simulink model "F16ASYM_Controlled"  (R2015a)
settings: Solver=ode3  SolverMode=SingleTasking  StartTime=0.0  StopTime=inf  FixedStep=T_sim  RelTol=1e-3
InitFcn:
  | load('NN_c_weights_Last_stable.mat')
StopFcn:
  | Final_results
values from neighbouring files (symbols this model uses):
  a1 = fitresult.p1    [Stall_protection.m]
  alpha_map_eval = ones(size(M_eval))*NaN    [Auto_trim_aid.m]    (also in Autotrim_maps.mat = [nan nan 0.277598136245 0.119432432992 0.0579479097061 0.027)
  beta_map_eval = ones(size(M_eval))*NaN    [Auto_trim_aid.m]    (also in Autotrim_maps.mat = [nan nan -0.00151549403324 0.00117807579006 -0.0052086799721)
  C_L_0 = fitresult.p2    [Stall_protection.m]
  G_eval = NaN*ones(size(M_sq,2),size(H_sq,2))    [Stall_protection.m]
  H_sq = unique(sort(H_sq))    [Stall_protection.m]
  H_sq_autotrim = min( F_envelope.H_1g):2000:max(F_envelope.H_1g)    [Auto_trim_aid.m]    (also in Autotrim_maps.mat = [0 2000 4000 6000 8000 10000 12000 14000 16000 18000])
  K_b_q_extrap_ACC = K_b_q_extrap    [RUN_ME.m]
  K_b_q_extrap_AoA = K_b_q_extrap    [RUN_ME.m]
  M_sq = unique(sort(M_sq))    [Stall_protection.m]
  M_sq_autotrim = 0:0.1:max(F_envelope.M_1g)    [Auto_trim_aid.m]    (also in Autotrim_maps.mat = [0 0.1 0.2 0.3 0.4 0.5 0.6 0.7 0.8 0.9 1 1.1 ... (21 element)
  T_sim = 0.02    [RUN_ME.m]
  tau_q_extrap_ACC = tau_q_extrap    [RUN_ME.m]
  tau_q_extrap_AoA = tau_q_extrap    [RUN_ME.m]
  velocity = M_eval(I,J)*a    [Auto_trim_aid.m]
undefined symbols (not defined in the file or in its folder): ACCEL, B, Earth, fi_flag_Simulink, GYRO, H_sq_sche, k_B, K_b_ACC_extrap, K_b_AoA_extrap, latitude, longitude, m, m_B, M_sq_sche, Model_used_flag, rad, s, sigbuilder_block, Stall_curve, tau_ACC_extrap, tau_AoA_extrap, Theta_1_roll_last, Theta_2_roll_last, Theta_3_roll_last, trim_control, trim_state, trim_throttle, V_Comp_A_w_z_last, V_Comp_last, V_Comp_last_ONE, V_long_lastA_w_z, V_long_lastAoA, V_roll_last, V_roll_lastMOD, V_yaw_last, W_Comp_A_w_z_last, W_Comp_last, W_long_lastA_w_z, W_long_lastAoA, W_roll_last, W_roll_lastMOD, W_yaw_last, WGS84
libraries: Adaptive_FaultTolerantControl x57, dspsigops x37, F16_Actuator_Library x14, commnoisgen2 x13, simulink x11, simulink_extras x10, dsparch4 x6, aerolibatmos2 x6, aerolibtransform2 x6, aerolibfltsims x3, dspvision x3, dspsnks4 x3
(part 2 of 14)

== system F16ASYM_Controlled/Plotting ==
  States : Inport
  Demmands : Inport  Port=2
  Control Defl : Inport  Port=3
  Ailerons : Scope  NumInputPorts=3
      settings: ShowLegends=on  TimeRange=25  YMin=0~0.04~-0.249  YMax=0.045~0.065~-0.231  SaveName=ScopeData6  Decimation=2
  Attitude : Scope  NumInputPorts=3
      settings: TimeRange=50  YMin=0.41~13.75~0.675  YMax=0.5~14.5~1.025  SaveName=EULER_PLOT  Decimation=2  SampleTime=0.001
  Demux : Demux  Outputs=5
  Demux1 : Demux  Outputs=20
  Demux2 : Demux  Outputs=7
  LEFs : Scope  NumInputPorts=2
      settings: ShowLegends=on  TimeRange=10  YMin=24.9965~-0.05  YMax=25.001~1.05  SaveName=ScopeData10  Decimation=2
  Load factors : Scope  NumInputPorts=3
      settings: YMin=-0.022~0.000572~0.999425  YMax=-0.0195~0.000579~0.999775  SaveName=ScopeData4  Decimation=20
  Mux{1..5} (5 alike) : Mux  Inputs=2
  Mux6 : Mux  Commented=on  Inputs=2
  Mux7 : Mux  Inputs=5
  Mux8 : Mux  Commented=on  Inputs=3
  "POW, Mach, q, ps" : Scope  NumInputPorts=4
      settings: YMin=-5~-5~-5~-5  YMax=5~5~5~5  SaveName=ScopeData5  Decimation=20
  Responses and commands : Scope  NumInputPorts=5
      settings: ShowLegends=on  TimeRange=50  YMin=1~11.6575~-0.04~-0.525~75  YMax=14~11.675~0.06~-0.325~125  SaveName=Responses  Decimation=2
  To Workspace : ToWorkspace  Commented=on  VariableName=DR1  SaveFormat=Timeseries  SampleTime=-1
  To Workspace1 : ToWorkspace  VariableName=Control_defl  SaveFormat=Timeseries  SampleTime=-1
  To Workspace2 : ToWorkspace  VariableName=Responses_out  SaveFormat=Timeseries  SampleTime=-1
  To Workspace3 : ToWorkspace  VariableName=ALL_Responses_out  SaveFormat=Timeseries  SampleTime=-1
  To Workspace4 : ToWorkspace  Commented=on  VariableName=SPPO4_ge  SaveFormat=Timeseries  SampleTime=-1
  To Workspace5 : ToWorkspace  Commented=on  VariableName=ROLL  SaveFormat=Timeseries  SampleTime=-1
  elevs : Scope  NumInputPorts=2
      settings: ShowLegends=on  TimeRange=10  YMin=-2.7018~-2.678  YMax=-2.6998~-2.67525  SaveName=ScopeData9  Decimation=2
  p,q,r : Scope  NumInputPorts=3
      settings: TimeRange=15  YMin=-3~-0.04~-3  YMax=7~0.04~9  SaveName=ScopeData3  Decimation=2
  position and altitude : Scope  NumInputPorts=3
      settings: YMin=12100~6e-11~13235  YMax=13700~8.75e-11~13320  Decimation=20
  wires:
  Demux1/1 -> position and altitude/1  "npos   (m)"
  Demux1/2 -> position and altitude/2  "epos   (m)"
  Demux1/3 -> position and altitude/3  "alt   (m)"
  Demux1/5 -> Attitude/2  "theta   (deg)"
  Demux1/6 -> Attitude/3  "psi  (deg)"
  Demux1/7 -> Mux5/2  "TAS   (m/s)"
  Demux1/8 -> Mux1/2  "alpha( deg)"
  Demux1/9 -> Mux3/2  "beta  (deg)"
  Demux1/10 -> To Workspace5/1, Mux6/1, p,q,r/1, Mux2/2  "p   (deg/s)"
  Demux1/11 -> Mux8/3, p,q,r/2  "q   (deg/s)"
  Demux1/12 -> Mux6/2, p,q,r/3  "r   (deg/s)"
  Demux1/14 -> Load factors/1  "nx (g)"
  Demux1/15 -> Load factors/2  "ny (g)"
  Demux1/16 -> Load factors/3  "nz (g)"
  Demux1/4 -> Attitude/1  "phi   (deg)"
  Demux1/17 -> "POW, Mach, q, ps"/2  "mach"
  Demux1/18 -> "POW, Mach, q, ps"/3  "qbar (Pa"
  Demux1/19 -> "POW, Mach, q, ps"/4  "ps (Pa)"
  States/1 -> To Workspace3/1, Demux1/1
  Demux1/13 -> "POW, Mach, q, ps"/1  "pow"
  Demmands/1 -> Demux/1
  Mux2/1 -> Mux7/3, Responses and commands/3
  Mux3/1 -> Mux7/4, Responses and commands/4
  Demux/2 -> Mux1/1  "alpha comm"
  Demux/3 -> Mux2/1  "p comm"
  Demux/4 -> Mux3/1  "beta comm"
  Mux4/1 -> Mux8/1, Mux7/1, Responses and commands/1
  Demux/1 -> Mux4/1  "A_w_z comm"
  Demux1/20 -> Mux4/2  "A_w_z (m/s^2)"
  Control Defl/1 -> To Workspace1/1, Demux2/1
  Demux2/3 -> Ailerons/1  "Aileron Left"
  Demux2/7 -> LEFs/2  "LEF Right"
  Demux2/6 -> LEFs/1  "LEF Left"
  Demux2/2 -> elevs/2  "Elevator_ Right"
  Demux2/5 -> Ailerons/3  "Rudder"
  Demux2/4 -> Ailerons/2  "Aielron Right"
  Mux5/1 -> Mux7/5, Responses and commands/5
  Demux/5 -> Mux5/1  "TAS comm"
  Mux1/1 -> Mux8/2, Mux7/2, Responses and commands/2
  Mux6/1 -> To Workspace/1
  Demux2/1 -> elevs/1  "Elevator_ Left"
  Mux7/1 -> To Workspace2/1
  Mux8/1 -> To Workspace4/1

== system F16ASYM_Controlled/Primary Controller ==
  A_w_z des : Inport
  AoA des (rad) : Inport  Port=2
  p des (rad/s) : Inport  Port=3
  beta des (rad) : Inport  Port=4
  Anti-windup A_w_z : Inport  Port=5
  Anti-windup AoA : Inport  Port=6
  Anti-windup beta : Inport  Port=7
  All measures : Inport  Port=8
  Anti-windup signals : Inport  Port=9
  P con  + Crossed NN + AWU+Lim + hand-over+Scheduling : Subsystem  VariantControl=Adaptive Controller Crossed+AWU+Lim+hand-over+Sched
  P con + Crossed NN + AWU+Lim + hand-over : Subsystem  VariantControl=Adaptive Controller Crossed+AWU+Lim+hand-over
  P con + adaptive Crossed NN + AWU+Lim + Scheduling : Subsystem  VariantControl=Adaptive Controller Crossed+AWU+Lim+Sched
  "P cont + adaptive Crossed NN + AWU+Lim " : Subsystem  VariantControl=Adaptive Controller Crossed+AWU+Lim
  P cont + adaptive Crossed NN + AWU+Lim ONELAYER : Subsystem  VariantControl=ONE
  P controller : Subsystem  VariantControl=P Controller
  P controller + adaptive Crossed NN : Subsystem  VariantControl=Adaptive Controller Crossed
  P controller + adaptive Isolated NN : Subsystem  VariantControl=Adaptive Controller Isolated
  PI Primary Controller : Subsystem  VariantControl=PI Controller
  Angular acc des : Outport
  Control_in : Outport  Port=2

== system F16ASYM_Controlled/SI and FDI ==
  Inexistent Reconfig bus : Inport
  Control comms : Inport  Port=2
  All  meas : Inport  Port=3
  SI and FDI: Realistic : Subsystem  VariantControl=Realistic
  SI and FDI: Unrealistic : Subsystem  VariantControl=Unrealistic
  Est reconf params : Outport

== system F16ASYM_Controlled/Sensors and filtering ==
  state : Inport
  Sensors and filtering. No noise : Subsystem  VariantControl=No noise
  Sensors and filtering. Noise : Subsystem  VariantControl=Noise
  All_measures : Outport

== system F16ASYM_Controlled/Signal Builder ==
  Demux : Demux  Tag=STV Demux  Outputs=1
  FromWs : FromWorkspace  Tag=STV FromWs  VariableName=tuvar  SampleTime=0
      SigBuilderData=|
      | common.afterFinalStr = 'Extrapolate'
      | common.sampleTime = 0
      | dataSet.timeRange = [0 10]
      | dataSet.name = 'Group 1'
      | sbobj.Groups.Name = 'Group 1'
      | sbobj.Groups.Signals.Name = 'Signal 1'
      | sbobj.Groups.Signals.XData = [0 8 8 8.5 8.5 10]
      | sbobj.Groups.Signals.YData = [0 0 0.51 0.51 0 0]
  Signal 1 : Outport  Tag=STV Outport
  wires:
  Demux/1 -> Signal 1/1
  FromWs/1 -> Demux/1

== system F16ASYM_Controlled/Speed-Throttle control ==
  All meas : Inport
  Throttle comm : Inport  Port=2
  delta TAS comm : Inport  Port=3
  "   " : Sum  Inputs=++|
  Add1 : Sum  Inputs=++|
  Manual Switch : ManualSwitch  CurrentSetting=0
  Stall protection TAS : Subsystem
  Throttle Trim Setting : Constant  Value=trim_throttle
  Throttle controller : Subsystem
  V_TAS des : Constant  Value=velocity
  Throttle des : Outport
  TAS des : Outport  Port=2
  wires:
  Throttle controller/1(Throttle des) -> Manual Switch/2
  Add1/1 -> Manual Switch/1
  Throttle Trim Setting/1 -> Add1/1
  Manual Switch/1 -> Throttle des/1
  Stall protection TAS/1(TAS des) -> Throttle controller/1(V_TAS des), TAS des/1
  Throttle comm/1 -> Add1/2
  delta TAS comm/1 -> "   "/2
  V_TAS des/1 -> "   "/1
  "   "/1 -> Stall protection TAS/1(TAS comm)
  All meas/1 -> Stall protection TAS/2(All meas), Throttle controller/2(All meas)

== system F16ASYM_Controlled/Stall protection A_z and AoA ==
  Control in : Inport
  Reconf param : Inport  Port=2
  All meas : Inport  Port=3
  A_w_z comm : Inport  Port=4
  AoA comm : Inport  Port=5
  AoA and load factor map : Subsystem  VariantControl=AoA and load factor
  Using AoA : Subsystem  VariantControl=Using AoA
  A_w_z des : Outport
  AoA des : Outport  Port=2

== system F16ASYM_Controlled/SubSystem3 ==

== system F16ASYM_Controlled/rad2deg ==
  note: npos,epos,alt
  note: phi
  note: theta
  note: psi
  note: v
  note: alpha
  note: beta
  note: p
  note: q
  note: r
  Params bus : Inport
  States Bus : Inport  Port=2
  Bus Selector : BusSelector  OutputSignals=States_out,Other outs
  Bus Selector1 : BusSelector  OutputSignals=A_w_CG
  Demux1 : Demux  Outputs=[3 1 1 1 1 1 1 1 1 1 1 3 3]
  Gain : Gain  Gain=-1
  Mux : Mux  Inputs=[3 1 1 1 1 1 1 1 1 1 1 3 3 1]
  Mux1 : Mux  Inputs=2
  Selector : Selector  InputPortWidth=3  Indices=3
  r2d{,1..7} (8 alike) : Gain  Gain=180/pi  SaturateOnIntegerOverflow=on  OutDataTypeStr=Inherit: Same as input  ParamDataTypeStr=Inherit: Same as input
  Out1 : Outport
  wires:
  Mux1/1 -> Demux1/1
  Demux1/2 -> r2d/1
  Demux1/3 -> r2d1/1
  Demux1/4 -> r2d2/1
  Demux1/1 -> Mux/1
  Demux1/5 -> Mux/5
  r2d2/1 -> Mux/4
  r2d1/1 -> Mux/3
  r2d/1 -> Mux/2
  Demux1/6 -> r2d3/1
  Demux1/7 -> r2d4/1
  Demux1/8 -> r2d5/1
  Demux1/9 -> r2d6/1
  Demux1/10 -> r2d7/1
  r2d4/1 -> Mux/7
  r2d5/1 -> Mux/8
  r2d6/1 -> Mux/9
  r2d7/1 -> Mux/10
  Mux/1 -> Out1/1
  Demux1/12 -> Mux/12  "nx,ny,nz"
  Demux1/13 -> Mux/13  "mach,qbar,ps"
  r2d3/1 -> Mux/6
  Demux1/11 -> Mux/11  "pow"
  Bus Selector/1 -> Mux1/1  "<States_out>"
  Bus Selector/2 -> Mux1/2  "<Other outs>"
  States Bus/1 -> Bus Selector/1
  Params bus/1 -> Bus Selector1/1
  Bus Selector1/1 -> Selector/1  "<A_w_CG>"
  Selector/1 -> Gain/1
  Gain/1 -> Mux/14

== system F16ASYM_Controlled/Anti-windup Calculation/Anti-windup: NO reconfigurable ==
  note: Reached Angular accel
  note: Converto to Angular accelerations
  Ang accel comm : Inport
  Est reconf : Inport  Port=2
  All_meas : Inport  Port=3
  Surf saturated : Inport  Port=4
  Control_defl : Inport  Port=5
  Analog Filter Design1 : dsparch4/Analog Filter Design  method=Butterworth  filttype=Lowpass  N=8  Wlo=2*pi/T_sim/4  Whi=80  Rp=2  Rs=40
  Analog Filter Design2 : dsparch4/Analog Filter Design  method=Butterworth  filttype=Lowpass  N=8  Wlo=2*pi/T_sim/4  Whi=80  Rp=2  Rs=40
  Analog Filter Design3 : dsparch4/Analog Filter Design  method=Butterworth  filttype=Lowpass  N=8  Wlo=2*pi/T_sim/4  Whi=80  Rp=2  Rs=40
  Ang Accel : MATLAB Function
  Antiwindup calculation : MATLAB Function  TreatAsAtomicUnit=on
  Bus Selector : BusSelector  OutputSignals=signal1.Alt meas (m),signal1.V_TAS (m/s),signal1.AoA meas (rad),signal1.SS meas (rad),signal1.omega_b meas (rad/s),signal1.Throttle_meas
  Bus Selector1 : BusSelector  OutputSignals=signal2.q (Pa),signal1.omega_b meas (rad/s)
  Demux : Demux  Outputs=3
  Demux1 : Demux  Outputs=3
  Effectiveness Matrix B : Constant  Value=B
  Memory1 : Memory  X0=[0,0,0]
  Mom coefficients that was reached : MATLABFcn  MATLABFcn=Moms_Coeff_estimator  OutputDimensions=3  OutputSignalType=real
  Moments : Subsystem
  Mux : Mux  Inputs=3
  Mux1 : Mux  Inputs=7
  Mux2 : Mux  Inputs=3
  Selector : Selector  InputPortWidth=8  Indices=1:7
  Terminator1 : Terminator
  Anti-windup signals : Outport
  wires:
  Selector/1 -> Antiwindup calculation/5(deflections), Mux1/7
  Mux1/1 -> Mom coefficients that was reached/1
  Bus Selector/5 -> Mux1/5  "<omega_b meas (rad/s)>"
  Bus Selector/1 -> Mux1/1  "<Alt meas (m)>"
  Bus Selector/2 -> Mux1/2  "<V_TAS (m/s)>"
  Bus Selector/3 -> Mux1/3  "<AoA meas (rad)>"
  Bus Selector/4 -> Mux1/4  "<SS meas (rad)>"
  Control_defl/1 -> Selector/1
  Bus Selector/6 -> Mux1/6  "<Throttle_meas>"
  Ang Accel/2(q_dot) -> Mux/2
  Ang Accel/3(r_dot) -> Mux/3
  Ang Accel/1(p_dot) -> Mux/1
  Bus Selector1/2 -> Ang Accel/4(omega_b)  "<omega_b meas (rad/s)>"
  Moments/3(N) -> Ang Accel/3(N)
  Moments/2(M) -> Ang Accel/2(M)
  Moments/1(L) -> Ang Accel/1(L)
  Bus Selector1/1 -> Moments/4(q)  "<q (Pa)>"
  Demux/3 -> Moments/3(C_N)
  Demux/2 -> Moments/2(C_M)
  Demux/1 -> Moments/1(C_L)
  Mom coefficients that was reached/1 -> Demux/1
  All_meas/1 -> Bus Selector/1, Bus Selector1/1
  Est reconf/1 -> Terminator1/1
  Mux/1 -> Antiwindup calculation/2(Ang_acell_achieved)
  Effectiveness Matrix B/1 -> Antiwindup calculation/4(B)
  Surf saturated/1 -> Antiwindup calculation/3(Saturations)
  Ang accel comm/1 -> Memory1/1
  Memory1/1 -> Antiwindup calculation/1(Ang_acell_comm)
  Mux2/1 -> Anti-windup signals/1
  Antiwindup calculation/1(AWU) -> Demux1/1
  Demux1/1 -> Analog Filter Design3/1
  Demux1/2 -> Analog Filter Design1/1
  Analog Filter Design3/1 -> Mux2/1
  Analog Filter Design1/1 -> Mux2/2
  Analog Filter Design2/1 -> Mux2/3
  Demux1/3 -> Analog Filter Design2/1

== system F16ASYM_Controlled/Anti-windup Calculation/Anti-windup: Reconfigurable ==
  note: INPUTS
      | States:
      |
      | 1. Altitude
      | 2. TAS velocity
      | 3. alpha in rad
      | 4. beta in rads
      | 5. P
      | 6. Q
      | 7. R
      | 8. Throttle
      | 9. Elevator_L in deg
      | 10. Elevator_R in deg
      | 11. Aileron_L
      | 12. Aileron_R
      | 13. Rudder
      | 14. LEF_L
      | 15. LEF_R
      |
      | RECONFIGURATION PARAMETERS
      |
      | 16. mass  Estimated mass
      | 17. S_current_L
      | 18. S_current_R
      | 19. S_fin_current
      | 20. x_cg
      | 21. Jy
      | 22. Jxz
      | 23. Jz
      | 24. Jx
      | 25. EFF_el_L
      | 26. EFF_el_R
      | 27. EFF_ail_L
      | 28 EFF_ail_R
      | 29. EFF_rud
      | 30. EFF_lef_L
      | 31. EFF_lef_R
      | 32. Delta_C_Lift_X
      | 33. Delta_C_Drag_X
      | 34. Delta_C_m_X
  note: Reached Angular accel
  note: Converto to Angular accelerations
  Ang accel comm : Inport
  Est reconf : Inport  Port=2
  All_meas : Inport  Port=3
  Surf saturated : Inport  Port=4
  Control_defl : Inport  Port=5
  Analog Filter Design1 : dsparch4/Analog Filter Design  method=Butterworth  filttype=Lowpass  N=8  Wlo=2*pi/T_sim/5  Whi=80  Rp=2  Rs=40
  Analog Filter Design2 : dsparch4/Analog Filter Design  method=Butterworth  filttype=Lowpass  N=8  Wlo=2*pi/T_sim/5  Whi=80  Rp=2  Rs=40
  Analog Filter Design3 : dsparch4/Analog Filter Design  method=Butterworth  filttype=Lowpass  N=8  Wlo=2*pi/T_sim/5  Whi=80  Rp=2  Rs=40
  Ang Accel : MATLAB Function
  Antiwindup calculation : MATLAB Function  TreatAsAtomicUnit=on
  Bus Selector : BusSelector  OutputSignals=signal1.Alt meas (m),signal1.V_TAS (m/s),signal1.AoA meas (rad),signal1.SS meas (rad),signal1.omega_b meas (rad/s),signal1.Throttle_meas
  Bus Selector1 : BusSelector  OutputSignals=signal2.q (Pa),signal1.omega_b meas (rad/s)
  Bus Selector2 : BusSelector  OutputSignals=Reconfig signal
  Demux : Demux  Outputs=3
  Demux1 : Demux  Outputs=3
  Effectiveness Matrix B : Constant  Value=B
  Memory1 : Memory  X0=[0,0,0]
  "Mom coefficients that was reached " : MATLABFcn  MATLABFcn=Moms_Coeff_Reconf_estimator  OutputDimensions=3  OutputSignalType=real
  Moments : Subsystem
  Mux : Mux  Inputs=3
  Mux1 : Mux  Inputs=7
  Mux2 : Mux  Inputs=3
  Mux3 : Mux  Inputs=[15 19]
  Selector : Selector  InputPortWidth=8  Indices=1:7
  Signal Specification : SignalSpecification  Dimensions=19
  Transfer Fcn1 : TransferFcn  Commented=on  Numerator=10  Denominator=[1 10]
  Anti-windup signals : Outport
  wires:
  Bus Selector/6 -> Mux1/6  "<Throttle_meas>"
  Control_defl/1 -> Selector/1
  Bus Selector/4 -> Mux1/4  "<SS meas (rad)>"
  Bus Selector/3 -> Mux1/3  "<AoA meas (rad)>"
  Bus Selector/2 -> Mux1/2  "<V_TAS (m/s)>"
  Bus Selector/1 -> Mux1/1  "<Alt meas (m)>"
  Bus Selector/5 -> Mux1/5  "<omega_b meas (rad/s)>"
  Selector/1 -> Antiwindup calculation/5(deflections), Mux1/7
  Est reconf/1 -> Bus Selector2/1
  Bus Selector2/1 -> Signal Specification/1  "<Reconfig signal>"
  Mux1/1 -> Mux3/1
  Mux3/1 -> "Mom coefficients that was reached "/1
  Signal Specification/1 -> Mux3/2
  All_meas/1 -> Bus Selector1/1, Bus Selector/1
  Ang Accel/2(q_dot) -> Mux/2
  Ang Accel/3(r_dot) -> Mux/3
  Ang Accel/1(p_dot) -> Mux/1
  Bus Selector1/2 -> Ang Accel/4(omega_b)  "<omega_b meas (rad/s)>"
  Moments/3(N) -> Ang Accel/3(N)
  Moments/2(M) -> Ang Accel/2(M)
  Moments/1(L) -> Ang Accel/1(L)
  Bus Selector1/1 -> Moments/4(q)  "<q (Pa)>"
  Demux/3 -> Moments/3(C_N)
  Demux/2 -> Moments/2(C_M)
  Demux/1 -> Moments/1(C_L)
  "Mom coefficients that was reached "/1 -> Demux/1
  Mux/1 -> Antiwindup calculation/2(Ang_acell_achieved)
  Effectiveness Matrix B/1 -> Antiwindup calculation/4(B)
  Surf saturated/1 -> Antiwindup calculation/3(Saturations)
  Ang accel comm/1 -> Memory1/1
  Memory1/1 -> Antiwindup calculation/1(Ang_acell_comm)
  Antiwindup calculation/1(AWU) -> Demux1/1
  Demux1/1 -> Analog Filter Design3/1
  Demux1/2 -> Analog Filter Design1/1
  Analog Filter Design3/1 -> Mux2/1
  Analog Filter Design1/1 -> Mux2/2
  Analog Filter Design2/1 -> Mux2/3
  Demux1/3 -> Analog Filter Design2/1
  Mux2/1 -> Anti-windup signals/1

== system F16ASYM_Controlled/Auto-trim, saturations sensibility and pilot help/Command A_w_z  or  A_gamma_z ==
  note: Pass this one if >0.5
  All meas : Inport
  Acc command : Inport  Port=2
  A_b : Product  Multiplication=Matrix(*)
  A_w : Product  Multiplication=Matrix(*)
  Bus Selector3 : BusSelector  OutputSignals=signal2.T_F_b->F_T,signal2.T_F_b->F_w
  Criteria : Constant  Value=Criteria
  Gain : Gain  Gain=[0;0;-1]
  Gain1 : Gain  Gain=-1
  Selector : Selector  InputPortWidth=3  Indices=3
  Switch : Switch  Threshold=0.5
  Transpose : Math  Operator=transpose  SaturateOnIntegerOverflow=on
  A_w_z : Outport
  wires:
  All meas/1 -> Bus Selector3/1
  Criteria/1 -> Switch/2
  Acc command/1 -> Switch/3, Gain/1
  Switch/1 -> A_w_z/1
  Bus Selector3/1 -> Transpose/1  "<T_F_b->F_T>"
  Transpose/1 -> A_b/1
  Gain/1 -> A_b/2
  Bus Selector3/2 -> A_w/1  "<T_F_b->F_w>"
  A_b/1 -> A_w/2
  A_w/1 -> Selector/1
  Selector/1 -> Gain1/1
  Gain1/1 -> Switch/1

== system F16ASYM_Controlled/Cockpit/Joystick ==
  Add1 : Sum
  Add2 : Sum
  Aileron : Selector  InputPortWidth=2
  Gain : Gain  Gain=0.01  OutDataTypeStr=double
  Gain{1..2,4,8} (4 alike) : Gain
  Gain3 : Gain  Gain=-1
  Gain5 : Gain  Gain=-1
  Gain6 : Gain  Gain=10  OutDataTypeStr=double
  Gain7 : Gain  Gain=-1
  Integrator Limited2 : Integrator  LimitOutput=on  UpperSaturationLimit=400  LowerSaturationLimit=-400
  Integrator Limited3 : Integrator  LimitOutput=on  UpperSaturationLimit=1  LowerSaturationLimit=-1
  Joystick Input : vrlib/Joystick Input  joyid=1  adjustports=on  forcefeed=off
  Manual Switch : ManualSwitch
  Selector1 : Selector  InputPortWidth=5  Indices=1:2
  Selector2 : Selector  InputPortWidth=5  Indices=3
  Selector3 : Selector  InputPortWidth=5  Indices=4:5
  Selector4 : Selector  InputPortWidth=10
  Selector5 : Selector  InputPortWidth=10  Indices=4
  Selector6 : Selector  InputPortWidth=10
  Selector7 : Selector  InputPortWidth=10  Indices=4
  Selector8 : Selector  InputPortWidth=10  Indices=8
  Terminator : Terminator
  elev : Selector  InputPortWidth=2  Indices=2
  speed des : Outport
  Throttle : Outport  Port=2
  Long: Acc : Outport  Port=3
  Roll : Outport  Port=4
  sideslip : Outport  Port=5
  Trim now : Outport  Port=6
  wires:
  Integrator Limited3/1 -> Throttle/1  "Throttle"
  Aileron/1 -> Gain1/1
  Manual Switch/1 -> Aileron/1, elev/1
  Joystick Input/1 -> Selector2/1, Selector3/1, Selector1/1
  Selector1/1 -> Manual Switch/1
  Selector3/1 -> Manual Switch/2
  Selector4/1 -> Gain3/1
  Selector5/1 -> Gain4/1
  Gain3/1 -> Add1/1
  Gain4/1 -> Add1/2
  Add1/1 -> Gain/1
  Gain/1 -> Integrator Limited3/1
  elev/1 -> Gain2/1
  Gain1/1 -> Roll/1
  Gain2/1 -> Long: Acc/1
  Selector2/1 -> Gain5/1
  Integrator Limited2/1 -> speed des/1  "Throttle"
  Joystick Input/2 -> Selector8/1, Selector5/1, Selector7/1, Selector6/1, Selector4/1
  Selector6/1 -> Gain7/1
  Selector7/1 -> Gain8/1
  Gain7/1 -> Add2/1
  Gain8/1 -> Add2/2
  Add2/1 -> Gain6/1
  Gain6/1 -> Integrator Limited2/1
  ? -> Terminator/1
  Selector8/1 -> Trim now/1
  Gain5/1 -> sideslip/1

== system F16ASYM_Controlled/Cockpit/Signal Builder ==
  Demux : Demux  Tag=STV Demux  Outputs=3
  FromWs : FromWorkspace  Tag=STV FromWs  VariableName=tuvar  SampleTime=0
      SigBuilderData=|
      | common.afterFinalStr = 'Extrapolate'
      | common.sampleTime = 0
      | dataSet.timeRange = [0 5]
      | dataSet.name = 'Group 1'
      | sbobj.Groups.Name = 'Group 1'
      | sbobj.Groups.Signals(1).Name = 'Signal 1'
      | sbobj.Groups.Signals(1).XData = [0 2 2 4.985 4.985 5]
      | sbobj.Groups.Signals(1).YData = [0 0 -0.1 -0.1 0 0]
      | sbobj.Groups.Signals(2).Name = 'Signal 2'
      | sbobj.Groups.Signals(2).XData = [0 2.5 2.5 4.985 4.985 5]
      | sbobj.Groups.Signals(2).YData = [0 0 0.5 0.5 0 0]
      | sbobj.Groups.Signals(3).Name = 'Signal 3'
      | sbobj.Groups.Signals(3).XData = [0 5]
      | sbobj.Groups.Signals(3).YData = [0 0]
      | sbobj.Groups.TimeRange = [0 5]
  Signal 1 : Outport  Tag=STV Outport
  Signal 2 : Outport  Tag=STV Outport  Port=2
  Signal 3 : Outport  Tag=STV Outport  Port=3
  wires:
  FromWs/1 -> Demux/1
  Demux/1 -> Signal 1/1
  Demux/2 -> Signal 2/1
  Demux/3 -> Signal 3/1

== system F16ASYM_Controlled/Cockpit/Signal Builder1 ==
  Demux : Demux  Tag=STV Demux  Outputs=3
  FromWs : FromWorkspace  Tag=STV FromWs  VariableName=tuvar  SampleTime=0
      SigBuilderData=|
      | common.afterFinalStr = 'Extrapolate'
      | common.sampleTime = 0
      | dataSet.timeRange = [0 5]
      | dataSet.name = 'Group 1'
      | sbobj.Groups.Name = 'Group 1'
      | sbobj.Groups.Signals(1).Name = 'Signal 1'
      | sbobj.Groups.Signals(1).XData = [0 0.001 0.001 3.495 3.495 5]
      | sbobj.Groups.Signals(1).YData = [0 0 0.1 0.1 0 0]
      | sbobj.Groups.Signals(2).Name = 'Signal 2'
      | sbobj.Groups.Signals(2).XData = [0 0.001 0.001 2.51 2.51 5]
      | sbobj.Groups.Signals(2).YData = [0 0 -0.5 -0.5 0 0]
      | sbobj.Groups.Signals(3).Name = 'Signal 3'
      | sbobj.Groups.Signals(3).XData = [0 5]
      | sbobj.Groups.Signals(3).YData = [0 0]
      | sbobj.Groups.TimeRange = [0 5]
  Signal 1 : Outport  Tag=STV Outport
  Signal 2 : Outport  Tag=STV Outport  Port=2
  Signal 3 : Outport  Tag=STV Outport  Port=3
  wires:
  Demux/3 -> Signal 3/1
  Demux/2 -> Signal 2/1
  Demux/1 -> Signal 1/1
  FromWs/1 -> Demux/1

== system F16ASYM_Controlled/Cockpit/Signal Builder2 ==
  Demux : Demux  Tag=STV Demux  Outputs=3
  FromWs : FromWorkspace  Tag=STV FromWs  VariableName=tuvar  SampleTime=0
      SigBuilderData=|
      | common.afterFinalStr = 'Extrapolate'
      | common.sampleTime = 0
      | dataSet.timeRange = [0 5]
      | dataSet.name = 'Group 1'
      | sbobj.Groups.Name = 'Group 1'
      | sbobj.Groups.Signals(1).Name = 'Signal 1'
      | sbobj.Groups.Signals(1).XData = [0 2 4.985 5]
      | sbobj.Groups.Signals(1).YData = [0 0 0 0]
      | sbobj.Groups.Signals(2).Name = 'Signal 2'
      | sbobj.Groups.Signals(2).XData = [0 2.5 2.5 4.985 4.985 5]
      | sbobj.Groups.Signals(2).YData = [0 0 0.5 0.5 0 0]
      | sbobj.Groups.Signals(3).Name = 'Signal 3'
      | sbobj.Groups.Signals(3).XData = [0 5]
      | sbobj.Groups.Signals(3).YData = [0 0]
      | sbobj.Groups.TimeRange = [0 5]
  Signal 1 : Outport  Tag=STV Outport
  Signal 2 : Outport  Tag=STV Outport  Port=2
  Signal 3 : Outport  Tag=STV Outport  Port=3
  wires:
  Demux/3 -> Signal 3/1
  Demux/2 -> Signal 2/1
  Demux/1 -> Signal 1/1
  FromWs/1 -> Demux/1

== system F16ASYM_Controlled/Cockpit/Signal Builder3 ==
  Demux : Demux  Tag=STV Demux  Outputs=3
  FromWs : FromWorkspace  Tag=STV FromWs  VariableName=tuvar  SampleTime=0
      SigBuilderData=|
      | common.afterFinalStr = 'Extrapolate'
      | common.sampleTime = 0
      | dataSet.timeRange = [0 5]
      | dataSet.name = 'Group 1'
      | sbobj.Groups.Name = 'Group 1'
      | sbobj.Groups.Signals(1).Name = 'Signal 1'
      | sbobj.Groups.Signals(1).XData = [0 0.001 0.001 3.495 3.495 5]
      | sbobj.Groups.Signals(1).YData = [0 0 0 0 0 0]
      | sbobj.Groups.Signals(2).Name = 'Signal 2'
      | sbobj.Groups.Signals(2).XData = [0 0.001 0.001 2.51 2.51 5]
      | sbobj.Groups.Signals(2).YData = [0 0 -0.5 -0.5 0 0]
      | sbobj.Groups.Signals(3).Name = 'Signal 3'
      | sbobj.Groups.Signals(3).XData = [0 5]
      | sbobj.Groups.Signals(3).YData = [0 0]
      | sbobj.Groups.TimeRange = [0 5]
  Signal 1 : Outport  Tag=STV Outport
  Signal 2 : Outport  Tag=STV Outport  Port=2
  Signal 3 : Outport  Tag=STV Outport  Port=3
  wires:
  FromWs/1 -> Demux/1
  Demux/1 -> Signal 1/1
  Demux/2 -> Signal 2/1
  Demux/3 -> Signal 3/1

== system F16ASYM_Controlled/Cockpit/Signal Builder4 ==
  Demux : Demux  Tag=STV Demux  Outputs=3
  FromWs : FromWorkspace  Tag=STV FromWs  VariableName=tuvar  SampleTime=0
      SigBuilderData=|
      | common.afterFinalStr = 'Extrapolate'
      | common.sampleTime = 0
      | dataSet.timeRange = [0 10]
      | dataSet.name = 'Group 1'
      | sbobj.Groups.Name = 'Group 1'
      | sbobj.Groups.Signals(1).Name = 'Signal 1'
      | sbobj.Groups.Signals(1).XData = [0 2 4.985 10]
      | sbobj.Groups.Signals(1).YData = [0 0 0 0]
      | sbobj.Groups.Signals(2).Name = 'Signal 2'
      | sbobj.Groups.Signals(2).XData = [0 2.5 2.5 9.99 9.99 10]
      | sbobj.Groups.Signals(2).YData = [0 0 0.5 0.5 0 0]
      | sbobj.Groups.Signals(3).Name = 'Signal 3'
      | sbobj.Groups.Signals(3).XData = [0 10]
      | sbobj.Groups.Signals(3).YData = [0 0]
  Signal 1 : Outport  Tag=STV Outport
  Signal 2 : Outport  Tag=STV Outport  Port=2
  Signal 3 : Outport  Tag=STV Outport  Port=3
  wires:
  Demux/3 -> Signal 3/1
  Demux/2 -> Signal 2/1
  Demux/1 -> Signal 1/1
  FromWs/1 -> Demux/1

== system F16ASYM_Controlled/Cockpit/Signal Builder5 ==
  Demux : Demux  Tag=STV Demux  Outputs=3
  FromWs : FromWorkspace  Tag=STV FromWs  VariableName=tuvar  SampleTime=0
      SigBuilderData=|
      | common.afterFinalStr = 'Extrapolate'
      | common.sampleTime = 0
      | dataSet.timeRange = [0 10]
      | dataSet.name = 'Group 1'
      | sbobj.Groups.Name = 'Group 1'
      | sbobj.Groups.Signals(1).Name = 'Signal 1'
      | sbobj.Groups.Signals(1).XData = [0 0.001 3.495 10]
      | sbobj.Groups.Signals(1).YData = [0 0 0 0]
      | sbobj.Groups.Signals(2).Name = 'Signal 2'
      | sbobj.Groups.Signals(2).XData = [0 0.001 0.001 7.47 7.47 10]
      | sbobj.Groups.Signals(2).YData = [0 0 -0.5 -0.5 0 0]
      | sbobj.Groups.Signals(3).Name = 'Signal 3'
      | sbobj.Groups.Signals(3).XData = [0 10]
      | sbobj.Groups.Signals(3).YData = [0 0]
  Signal 1 : Outport  Tag=STV Outport
  Signal 2 : Outport  Tag=STV Outport  Port=2
  Signal 3 : Outport  Tag=STV Outport  Port=3
  wires:
  FromWs/1 -> Demux/1
  Demux/1 -> Signal 1/1
  Demux/2 -> Signal 2/1
  Demux/3 -> Signal 3/1

== system F16ASYM_Controlled/Cockpit/Signal Builder6 ==
  Demux : Demux  Tag=STV Demux  Outputs=3
  FromWs : FromWorkspace  Tag=STV FromWs  VariableName=tuvar  SampleTime=0
      SigBuilderData=|
      | common.afterFinalStr = 'Extrapolate'
      | common.sampleTime = 0
      | dataSet.timeRange = [0 10]
      | dataSet.name = 'Group 1'
      | sbobj.Groups.Name = 'Group 1'
      | sbobj.Groups.Signals(1).Name = 'Signal 1'
      | sbobj.Groups.Signals(1).XData = [0 2 4.985 10]
      | sbobj.Groups.Signals(1).YData = [0 0 0 0]
      | sbobj.Groups.Signals(2).Name = 'Signal 2'
      | sbobj.Groups.Signals(2).XData = [0 2.5 2.5 9.99 9.99 10]
      | sbobj.Groups.Signals(2).YData = [0 0 0.5 0.5 0 0]
      | sbobj.Groups.Signals(3).Name = 'Signal 3'
      | sbobj.Groups.Signals(3).XData = [0 10]
      | sbobj.Groups.Signals(3).YData = [0 0]
  Signal 1 : Outport  Tag=STV Outport
  Signal 2 : Outport  Tag=STV Outport  Port=2
  Signal 3 : Outport  Tag=STV Outport  Port=3
  wires:
  Demux/3 -> Signal 3/1
  Demux/2 -> Signal 2/1
  Demux/1 -> Signal 1/1
  FromWs/1 -> Demux/1

== system F16ASYM_Controlled/Cockpit/Signal Builder7 ==
  Demux : Demux  Tag=STV Demux  Outputs=3
  FromWs : FromWorkspace  Tag=STV FromWs  VariableName=tuvar  SampleTime=0
      SigBuilderData=|
      | common.afterFinalStr = 'Extrapolate'
      | common.sampleTime = 0
      | dataSet.timeRange = [0 10]
      | dataSet.name = 'Group 1'
      | sbobj.Groups.Name = 'Group 1'
      | sbobj.Groups.Signals(1).Name = 'Signal 1'
      | sbobj.Groups.Signals(1).XData = [0 0.001 3.495 10]
      | sbobj.Groups.Signals(1).YData = [0 0 0 0]
      | sbobj.Groups.Signals(2).Name = 'Signal 2'
      | sbobj.Groups.Signals(2).XData = [0 0.001 0.001 7.47 7.47 10]
      | sbobj.Groups.Signals(2).YData = [0 0 -0.5 -0.5 0 0]
      | sbobj.Groups.Signals(3).Name = 'Signal 3'
      | sbobj.Groups.Signals(3).XData = [0 10]
      | sbobj.Groups.Signals(3).YData = [0 0]
  Signal 1 : Outport  Tag=STV Outport
  Signal 2 : Outport  Tag=STV Outport  Port=2
  Signal 3 : Outport  Tag=STV Outport  Port=3
  wires:
  FromWs/1 -> Demux/1
  Demux/1 -> Signal 1/1
  Demux/2 -> Signal 2/1
  Demux/3 -> Signal 3/1

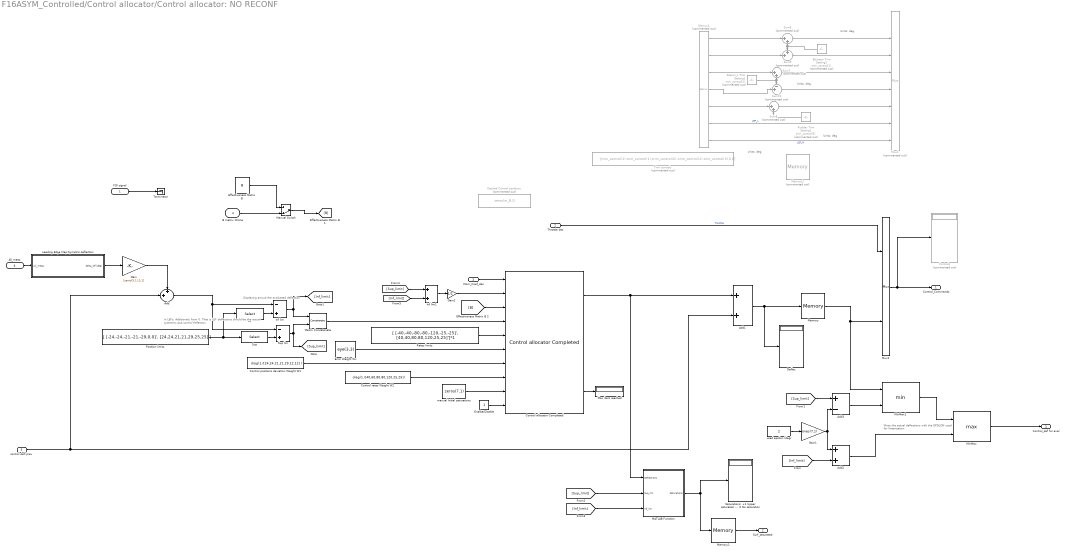
== system F16ASYM_Controlled/Control allocator/Control allocator: NO RECONF ==
  note: Wrap the actual deflections with the EPSILON
      |  used for linearization
  note: Units: deg.
  note: Units: deg.
  note: Units: deg.
  note: Units: deg.
  note: In LEFs: Additionaly from 0.  That is LEF deflections should be
      | the actual sytemtric AoA control felfection
  note: Displacing arroud the evaluated deflection
  FDI signal : Inport
  Throttle des : Inport  Port=2
  Mom_Coef_des : Inport  Port=3
  B matrix Online : Inport  Port=4
  control defl prev : Inport  Port=5
  All_meas : Inport  Port=6
  Add : Sum  Inputs=++|
  Add1 : Sum
  Add2 : Sum
  Add3 : Sum  Inputs=+-
  Aileron_L Trim Setting1 : Constant  Commented=on  Value=trim_control(2)
  "Control allocator Completed " : qcatlib/Control allocator Completed   alg=SLS  CA_type=QP  iter_max=100  gamma=1e6  k_B=3  m_B=7  T=T_sim  tol=1e-5
  Control positions deviation Weight W1 : Constant  Value=diag(1./[24,24,21,21,29,12,12] )
  Control rates Weight W2 : Constant  Value=diag(1./[40,60,80,80,120,25,25])
  Controls : Display  Commented=on
  Deflec : Display
  Demux1 : Demux  Commented=on  Outputs=[1,1,1,1,1,1,1]
  Desired Control positions : Constant  Commented=on  Value=zeros(m_B,1)
  Effectiveness Matrix B : Constant  Value=B
  Elevator Trim Setting1 : Constant  Commented=on  Value=trim_control(1)  VectorParams1D=off
  Enalbe/Disable : Constant
  Error Weight Wv : Constant  Value=eye(3,3)
  Gain : Gain  Gain=[zeros(5,1);1;1]
  Gain1 : Gain  Gain=ones(7,1)
  Gain2 : Gain  Gain=1/2
  Inf : Selector  NumberOfDimensions=2  InputPortWidth=3  IndexOptions=Index vector (dialog),Index vector (dialog)  Indices=[1:7],1  OutputSizes=1,1
  Inf lim : Sum  Inputs=-+
  Inf lim1 : Sum
  Leading Edge Flap:Symetric deflection : Subsystem
  MATLAB Function : MATLAB Function  TreatAsAtomicUnit=on
  Manual Switch : ManualSwitch  CurrentSetting=0
  Matrix Concatenate : Concatenate  Mode=Multidimensional array  ConcatenateDimension=2
  Max iters reached : Display
  Memory : Memory  X0=[trim_control(1),trim_control(1),trim_control(2),-trim_control(2),trim_control(3),0,0]'
  Memory1 : Memory  X0=zeros(7,1)
  Memory2 : Memory  Commented=on  X0=zeros(7,1)
  MinMax : MinMax  Function=max  Inputs=2
  MinMax1 : MinMax  Inputs=2
  Mux1 : Mux  Commented=on  Inputs=8
  Mux2 : Mux  Inputs=[1 7]
  Position limits : Constant  Value=[ [-24,-24,-21,-21,-29,0,0]', [24,24,21,21,29,25,25]']
  Rates limits : Constant  Value=[ [-40,-40,-80,-80,-120,-25,-25]', [40,40,80,80,120,25,25]']*1
  Rudder Trim Setting1 : Constant  Commented=on  Value=trim_control(3)
  Saturations: +1 Upper saturated -1 Lower saturated 0 No saturation : Display
  Sum10 : Sum  Commented=on  Inputs=-+|  SaturateOnIntegerOverflow=on  InputSameDT=on  OutDataTypeStr=Inherit: Same as first input
  Sum6 : Sum  Commented=on  Inputs=|++  SaturateOnIntegerOverflow=on  InputSameDT=on  OutDataTypeStr=Inherit: Same as first input
  Sum7 : Sum  Commented=on  Inputs=|++  SaturateOnIntegerOverflow=on  InputSameDT=on  OutDataTypeStr=Inherit: Same as first input
  Sum8 : Sum  Commented=on  Inputs=|++  SaturateOnIntegerOverflow=on  InputSameDT=on  OutDataTypeStr=Inherit: Same as first input
  Sum9 : Sum  Commented=on  Inputs=++|  SaturateOnIntegerOverflow=on  InputSameDT=on  OutDataTypeStr=Inherit: Same as first input
  Sup : Selector  NumberOfDimensions=2  InputPortWidth=3  IndexOptions=Index vector (dialog),Index vector (dialog)  Indices=[1:7],2  OutputSizes=1,1
  Sup lim : Sum  Inputs=-+
  Terminator : Terminator
  "Trim controls " : Constant  Commented=on  Value=[trim_control(1),trim_control(1),trim_control(2),-trim_control(2),trim_control(3),0,0]'
  manual Initial saturations : Constant  Value=zeros(7,1)
  used epsilon (deg) : Constant  Value=2
  Control_Commands : Outport
  Surf_saturated : Outport  Port=2
  Control_def for eval : Outport  Port=3
  wires:
  MinMax/1 -> Control_def for eval/1
  MinMax1/1 -> MinMax/1
  Add3/1 -> MinMax1/2
  used epsilon (deg)/1 -> Gain1/1
  [Inf_limit] -> Add2/2
  Gain1/1 -> Add3/2, Add2/1
  [Sup_limit] -> Add3/1
  Add2/1 -> MinMax/2
  Memory/1 -> Mux2/2, MinMax1/1
  Add1/1 -> Memory/1, Deflec/1
  Demux1/5 -> Sum8/1
  Rudder Trim Setting1/1 -> Sum8/2
  Elevator Trim Setting1/1 -> Sum9/1, Sum6/2
  Demux1/4 -> Sum10/2
  Demux1/3 -> Sum7/1
  Demux1/2 -> Sum9/2
  Demux1/1 -> Sum6/1
  Demux1/7 -> Mux1/8  "LEF_R"
  Demux1/6 -> Mux1/7  "LEF_L"
  Sum9/1 -> Mux1/3
  Sum6/1 -> Mux1/2
  Aileron_L Trim Setting1/1 -> Sum10/1, Sum7/2
  Sum10/1 -> Mux1/5
  Sum8/1 -> Mux1/6
  Sum7/1 -> Mux1/4
  ? -> Mux1/1  "Throttle"
  Control positions deviation Weight W1/1 -> "Control allocator Completed "/7
  FDI signal/1 -> Terminator/1
  Leading Edge Flap:Symetric deflection/1(delta_lef (deg)) -> Gain/1
  All_meas/1 -> Leading Edge Flap:Symetric deflection/1(All_meas)
  Gain/1 -> Add/1
  control defl prev/1 -> Add1/2, Add/2
  Manual Switch/1 -> [B]
  Effectiveness Matrix B/1 -> Manual Switch/1
  B matrix Online/1 -> Manual Switch/2
  "Control allocator Completed "/1 -> MATLAB Function/1(Deflections), Add1/1
  Enalbe/Disable/1 -> "Control allocator Completed "/10
  manual Initial saturations/1 -> "Control allocator Completed "/9
  "Control allocator Completed "/3 -> Max iters reached/1
  [B] -> "Control allocator Completed "/3
  Sup lim/1 -> [Sup_limit], Matrix Concatenate/2
  Inf lim/1 -> [Inf_limit], Matrix Concatenate/1
  Matrix Concatenate/1 -> "Control allocator Completed "/4
  Inf/1 -> Inf lim/2
  Add/1 -> Inf lim/1, Sup lim/1
  Sup/1 -> Sup lim/2
  Control rates Weight W2/1 -> "Control allocator Completed "/8
  Error Weight Wv/1 -> "Control allocator Completed "/6
  Rates limits/1 -> "Control allocator Completed "/5
  Position limits/1 -> Sup/1, Inf/1
  Gain2/1 -> "Control allocator Completed "/2
  Mux2/1 -> Control_Commands/1, Controls/1
  Throttle des/1 -> Mux2/1  "Throttle"
  Mom_Coef_des/1 -> "Control allocator Completed "/1
  [Sup_limit] -> MATLAB Function/2(Sup_lim)
  [Inf_limit] -> MATLAB Function/3(Inf_lim)
  MATLAB Function/1(Saturations) -> Memory1/1, Saturations: +1 Upper saturated -1 Lower saturated 0 No saturation/1
  [Sup_limit] -> Inf lim1/1
  [Inf_limit] -> Inf lim1/2
  Inf lim1/1 -> Gain2/1
  Memory1/1 -> Surf_saturated/1

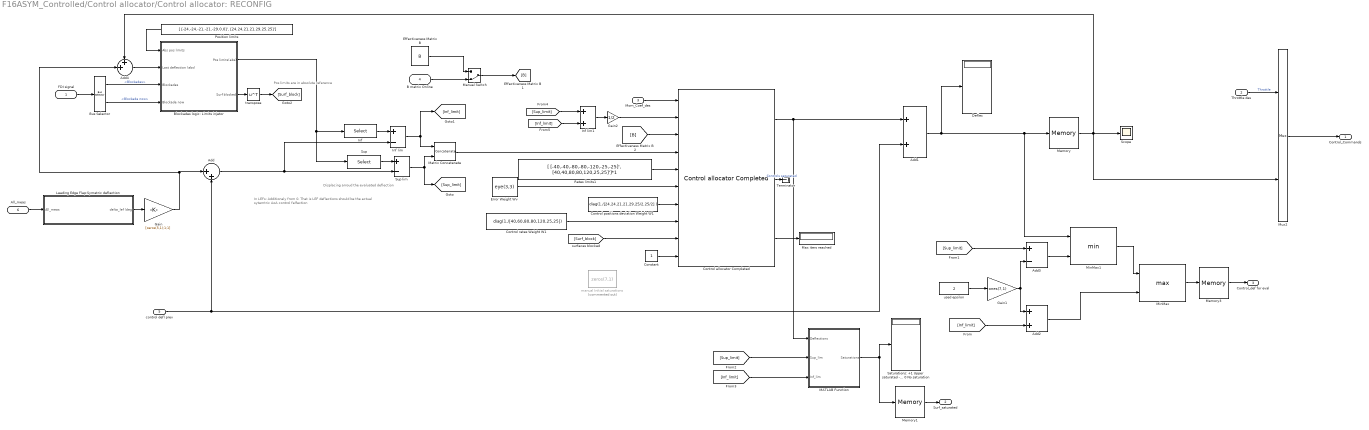
== system F16ASYM_Controlled/Control allocator/Control allocator: RECONFIG ==
  note: Pos limits are in absolute reference
  note: In LEFs: Additionaly from 0.  That is LEF deflections should be
      | the actual sytemtric AoA control felfection
  note: Displacing arroud the evaluated deflection
  FDI signal : Inport
  Throttle des : Inport  Port=2
  Mom_Coef_des : Inport  Port=3
  B matrix Online : Inport  Port=4
  control defl prev : Inport  Port=5
  All_meas : Inport  Port=6
  Add : Sum  Inputs=|++
  Add1 : Sum  SampleTime=T_sim
  Add2 : Sum
  Add3 : Sum  Inputs=+-
  Add4 : Sum  Inputs=++|
  Blockades logic: Limits injetor : Subsystem
  Bus Selector : BusSelector  OutputSignals=Blockades,Blockade now
  Constant : Constant
  "Control allocator Completed " : qcatlib/Control allocator Completed   alg=WLS  CA_type=QP  iter_max=100  gamma=1e8  k_B=3  m_B=7  T=T_sim  tol=1e-5
  Control positions deviation Weight W1 : Constant  Value=diag(1./[24,24,21,21,29,25/2,25/2] )
  Control rates Weight W1 : Constant  Value=diag(1./[40,60,80,80,120,25,25])
  Deflec : Display
  Effectiveness Matrix B : Constant  Value=B
  Error Weight Wv : Constant  Value=eye(3,3)
  Gain : Gain  Gain=[zeros(5,1);1;1]
  Gain1 : Gain  Gain=ones(7,1)
  Gain2 : Gain  Gain=1/2
  Inf : Selector  NumberOfDimensions=2  InputPortWidth=3  IndexOptions=Index vector (dialog),Index vector (dialog)  Indices=[1:7],1  OutputSizes=1,1
  Inf lim : Sum  Inputs=+-
  Inf lim1 : Sum
  Leading Edge Flap:Symetric deflection : Subsystem
  MATLAB Function : MATLAB Function  TreatAsAtomicUnit=on
  Manual Switch : ManualSwitch  CurrentSetting=0
  Matrix Concatenate : Concatenate  Mode=Multidimensional array  ConcatenateDimension=2
  Max iters reached : Display
  Memory : Memory  X0=[trim_control(1),trim_control(1),trim_control(2),-trim_control(2),trim_control(3),0,0]'  InheritSampleTime=on
  Memory1 : Memory  X0=zeros(7,1)
  Memory3 : Memory  X0=[trim_control(1),trim_control(1),trim_control(2),-trim_control(2),trim_control(3),0,0]'  InheritSampleTime=on
  MinMax : MinMax  Function=max  Inputs=2
  MinMax1 : MinMax  Inputs=2
  Mux2 : Mux  Inputs=[1 7]
  Position limits : Constant  Value=[ [-24,-24,-21,-21,-29,0,0]', [24,24,21,21,29,25,25]']
  Rates limits1 : Constant  Value=[ [-40,-40,-80,-80,-120,-25,-25]', [40,40,80,80,120,25,25]']*1
  Saturations: +1 Upper saturated -1 Lower saturated 0 No saturation : Display
  Scope : Scope
      settings: YMin=-25  YMax=20  SaveName=ScopeData22
  Sup : Selector  NumberOfDimensions=2  InputPortWidth=3  IndexOptions=Index vector (dialog),Index vector (dialog)  Indices=[1:7],2  OutputSizes=1,1
  Sup lim : Sum  Inputs=+-
  Terminator : Terminator
  manual Initial saturations : Constant  Commented=on  Value=zeros(7,1)
  transpose : Math  Operator=transpose  SaturateOnIntegerOverflow=on
  used epsilon : Constant  Value=2
  Control_Commands : Outport
  Surf_saturated : Outport  Port=2
  Control_def for eval : Outport  Port=3
  wires:
  Mom_Coef_des/1 -> "Control allocator Completed "/1
  Throttle des/1 -> Mux2/1  "Throttle"
  Mux2/1 -> Control_Commands/1
  Rates limits1/1 -> "Control allocator Completed "/5
  Error Weight Wv/1 -> "Control allocator Completed "/6
  Control rates Weight W1/1 -> "Control allocator Completed "/8
  Sup/1 -> Sup lim/1
  Add/1 -> Inf lim/2, Sup lim/2
  Inf/1 -> Inf lim/1
  Matrix Concatenate/1 -> "Control allocator Completed "/4
  [B] -> "Control allocator Completed "/3
  "Control allocator Completed "/3 -> Max iters reached/1
  [Surf_block] -> "Control allocator Completed "/9
  Constant/1 -> "Control allocator Completed "/10
  B matrix Online/1 -> Manual Switch/2
  Effectiveness Matrix B/1 -> Manual Switch/1
  control defl prev/1 -> Add1/2, Add/2
  Gain/1 -> Add/1, Add4/2
  All_meas/1 -> Leading Edge Flap:Symetric deflection/1(All_meas)
  Leading Edge Flap:Symetric deflection/1(delta_lef (deg)) -> Gain/1
  Control positions deviation Weight W1/1 -> "Control allocator Completed "/7
  Add1/1 -> Deflec/1, MinMax1/1, Memory/1
  Add2/1 -> MinMax/2
  Gain1/1 -> Add2/1, Add3/2
  used epsilon/1 -> Gain1/1
  Add3/1 -> MinMax1/2
  MinMax1/1 -> MinMax/1
  MinMax/1 -> Memory3/1
  Bus Selector/1 -> Blockades logic: Limits injetor/3(Blockades)  "<Blockades>"
  Bus Selector/2 -> Blockades logic: Limits injetor/4(Blockade now)  "<Blockade now>"
  FDI signal/1 -> Bus Selector/1
  Add4/1 -> Blockades logic: Limits injetor/2(Last deflection (abs))
  Position limits/1 -> Blockades logic: Limits injetor/1(Abs pos limits)
  Manual Switch/1 -> [B]
  [Sup_limit] -> Inf lim1/1
  [Inf_limit] -> Inf lim1/2
  Inf lim1/1 -> Gain2/1
  Gain2/1 -> "Control allocator Completed "/2
  "Control allocator Completed "/1 -> Add1/1, MATLAB Function/1(Deflections)
  [Sup_limit] -> MATLAB Function/2(Sup_lim)
  [Inf_limit] -> MATLAB Function/3(Inf_lim)
  MATLAB Function/1(Saturations) -> Memory1/1, Saturations: +1 Upper saturated -1 Lower saturated 0 No saturation/1
  Memory1/1 -> Surf_saturated/1
  "Control allocator Completed "/2 -> Terminator/1  "Controls saturated"
  Memory/1 -> Mux2/2, Scope/1, Add4/1
  Blockades logic: Limits injetor/2(Surf blocked) -> transpose/1
  transpose/1 -> [Surf_block]
  Sup lim/1 -> [Sup_limit], Matrix Concatenate/2
  Inf lim/1 -> [Inf_limit], Matrix Concatenate/1
  [Inf_limit] -> Add2/2
  [Sup_limit] -> Add3/1
  Memory3/1 -> Control_def for eval/1
  Blockades logic: Limits injetor/1(Pos limits(abs)) -> Inf/1, Sup/1

== system F16ASYM_Controlled/Environment params Estimations/Mach number ==
  V : Inport
  a : Inport  Port=2
  Product1 : Product  Inputs=*/  SaturateOnIntegerOverflow=on  InputSameDT=on  OutDataTypeStr=Inherit: Same as first input
  Mach : Outport
  wires:
  Product1/1 -> Mach/1
  V/1 -> Product1/1
  a/1 -> Product1/2

== system F16ASYM_Controlled/F-16 Non-linear Plant/SYM and ASYM model: No reconfigurable ==
  note: Mdoel used  Flage tells the plant
      |  if Asymetric or symetric model is used:
      | 0: Symetric Model
      | 1: Asymetric model
  note: INPUTS
      | States:
      | 1. North Position
      | 2. East position
      | 3. Altitude
      | 4. Phi
      | 5. Theta
      | 6. Psi
      | 7. Total velocity
      | 8. alpha in rad
      | 9. beta in rads
      | 10. P
      | 11. Q
      | 12. R
      | 13. POW
      |
      | Controls:
      | 14. Throttle
      | 15. Elevator_L in deg
      | 16. Elevator_R in deg
      | 17. Aileron_L
      | 18. Aileron_R
      | 19. Rudder
      | 20. LEF_L
      | 21. LEF_R
      |
      | 22. Fidelity Flag
      |
      | 23. Model used: Asymetric or Symetric
  note: Fidelity Flage tells nlplant
      | which Model to use:
      | 0: Low Fidelity
      | 1: High Fidelity
  note: OUTPUTS
      | States:
      | 1. DEV North Position
      | 2. DEV East position
      | 3. DEV Altitude
      | 4.DEV  Phi
      | 5. DEV Theta
      | 6. DEV Psi
      | 7. DEV Total velocity
      | 8.DEV alpha in rad
      | 9.DEV  beta in rads
      | 10. DEV P
      | 11. DEV Q
      | 12. DEV R
      | 13. DEV POW
      |
      | Other outputs:
      | Accels of CG:
      | 14. anx_cg
      | 15. any_cg
      | 16. anz_cg
      | 17. mach
      | 18. qbar
      | 19. ps   Static Pressure
  note: Add the sytmetric deflection of the LEFs
  States : Inport
  Reconf params : Inport  Port=2
  Control Comands : Inport  Port=3
  Acels actual : Scope
      settings: YMin=-0.04  YMax=0.09  SaveName=ScopeData14
  Actuators Dynamcis : Subsystem  TreatAsAtomicUnit=on
  Bus Creator : BusCreator  Inputs=12
  Bus Creator1 : BusCreator  Inputs=2
  Demux : Demux  Outputs=[13 6]
  Demux1 : Demux  Outputs=8
  F16 nlsim nlplant Asymetrical : MATLABFcn  MATLABFcn=nlplantASYM  OutputDimensions=19  OutputSignalType=real
  Fidelity Flag : Constant  Value=fi_flag_Simulink
  Integrate F16 State Derivatives : Integrator  InitialCondition=trim_state
  Leading Edge Flap:Symetric deflection : Subsystem
  Model used flag : Constant  Value=Model_used_flag
  Mux1 : Mux  Inputs=8
  Mux5 : Mux  Inputs=[13 8 1 1]
  Rotation Angles to Direction Cosine Matrix : aerolibtransform2/Rotation Angles to Direction Cosine Matrix  rotationOrder=ZYX
  Selector : Selector  InputPortWidth=13  Indices=[1:3]
  Selector1 : Selector  InputPortWidth=13  Indices=[1:3]
  Selector2 : Selector  InputPortWidth=13  Indices=[7]
  Selector3 : Selector  InputPortWidth=13  Indices=[8:9]
  Selector4 : Selector  InputPortWidth=13  Indices=[10:12]
  Selector5 : Selector  InputPortWidth=13  Indices=[4:6]
  Selector6 : Selector  InputPortWidth=6  Indices=[1:3]
  Selector7 : Selector  InputPortWidth=3  Indices=[3 2 1]
  Selector9 : Selector  InputPortWidth=13  Indices=[10:12]
  Sum1 : Sum  Inputs=|++  SaturateOnIntegerOverflow=on  InputSameDT=on  OutDataTypeStr=Inherit: Same as first input
  Sum9 : Sum  Inputs=|++  SaturateOnIntegerOverflow=on  InputSameDT=on  OutDataTypeStr=Inherit: Same as first input
  Output_bus : Outport
  Actual control def : Outport  Port=2
  wires:
  Selector7/1 -> Rotation Angles to Direction Cosine Matrix/1
  Demux/2 -> Bus Creator/3, Selector6/1  "Other outs"
  Selector6/1 -> Bus Creator/11  "an_b_CG"
  Selector5/1 -> Bus Creator/9, Selector7/1  "euler"
  Selector4/1 -> Bus Creator/8  "p,q,r"
  Selector3/1 -> Bus Creator/7  "alpha,beta"
  Selector2/1 -> Bus Creator/6  "TAS"
  Selector1/1 -> Bus Creator/5  "V_e"
  Selector/1 -> Bus Creator/4  "X_e"
  Demux/1 -> Integrate F16 State Derivatives/1, Selector1/1, Bus Creator/1, Selector9/1  "States_dot_out"
  Actuators Dynamcis/3(Throttle_meas) -> Bus Creator/12  "Throttle"
  Selector9/1 -> Acels actual/1
  Mux1/1 -> Actuators Dynamcis/1(Control_commands)
  Sum1/1 -> Mux1/8
  Sum9/1 -> Mux1/7
  Demux1/6 -> Mux1/6
  Demux1/4 -> Mux1/4
  Demux1/2 -> Mux1/2
  Demux1/1 -> Mux1/1
  Demux1/3 -> Mux1/3
  Demux1/5 -> Mux1/5
  Demux1/7 -> Sum9/1
  Demux1/8 -> Sum1/1
  Model used flag/1 -> Mux5/4
  F16 nlsim nlplant Asymetrical/1 -> Demux/1  "OUTPUTS"
  Mux5/1 -> F16 nlsim nlplant Asymetrical/1  "INPUTS"
  States/1 -> Mux5/1
  Control Comands/1 -> Demux1/1
  Fidelity Flag/1 -> Mux5/3
  Bus Creator/1 -> Leading Edge Flap:Symetric deflection/1(state), Output_bus/1
  Rotation Angles to Direction Cosine Matrix/1 -> Bus Creator/10  "DCM_b"
  Integrate F16 State Derivatives/1 -> Bus Creator/2, Selector/1, Selector2/1, Selector3/1, Selector4/1, Selector5/1  "States_out"
  Actuators Dynamcis/2(Dec_Control_def) -> Mux5/2
  Leading Edge Flap:Symetric deflection/1(delta_lef (deg)) -> Bus Creator1/1, Sum1/2, Sum9/2  "Symetric_LEF_defl"
  Bus Creator1/1 -> Actual control def/1
  Actuators Dynamcis/1(Control Defl Plot) -> Bus Creator1/2  "actual_control_defl"

== system F16ASYM_Controlled/F-16 Non-linear Plant/SYM and ASYM model: RECONFIGURABLE ==
  note: Add the sytmetric
      |  deflection of the LEFs
  note: OUTPUTS
      | States:
      | 1. DEV North Position
      | 2. DEV East position
      | 3. DEV Altitude
      | 4.DEV  Phi
      | 5. DEV Theta
      | 6. DEV Psi
      | 7. DEV Total velocity
      | 8.DEV alpha in rad
      | 9.DEV  beta in rads
      | 10. DEV P
      | 11. DEV Q
      | 12. DEV R
      | 13. DEV POW
      |
      | Other outputs:
      | Accels of CG:
      | 14. anx_cg
      | 15. any_cg
      | 16. anz_cg
      | 17. mach
      | 18. qbar
      | 19. ps   Static Pressure
  note: Fidelity Flage tells nlplant
      | which Model to use:
      | 0: Low Fidelity
      | 1: High Fidelity
  note: INPUTS
      | States:
      | 1. North Position
      | 2. East position
      | 3. Altitude
      | 4. Phi
      | 5. Theta
      | 6. Psi
      | 7. Total velocity
      | 8. alpha in rad
      | 9. beta in rads
      | 10. P
      | 11. Q
      | 12. R
      | 13. POW
      |
      | Controls:
      |
      | 14. Throttle
      | 15. Elevator_L in deg
      | 16. Elevator_R in deg
      | 17. Aileron_L
      | 18. Aileron_R
      | 19. Rudder
      | 20. LEF_L
      | 21. LEF_R
      |
      | 22. Fidelity Flag
      |
      | 23. Model used: Asymetric or Symetric
      |
      | RECONFIGURATION PARAMETERS
      |
      | 24. mass  Estimated mass
      | 25. S_current_L
      | 26. S_current_R
      | 27. S_fin_current
      | 28. x_cg
      | 29. Jy
      | 30. Jxz
      | 31. Jz
      | 32. Jx
      | 33. EFF_el_L
      | 34. EFF_el_R
      | 35. EFF_ail_L
      | 36. EFF_ail_R
      | 37. EFF_rud
      | 38. EFF_lef_L
      | 39. EFF_lef_R
      | 40. Delta_C_Lift_X
      | 41. Delta_C_Drag_X
      | 42. Delta_C_m_X
  note: Mdoel used  Flage tells the plant
      |  if Asymetric or symetric model is used:
      | 0: Symetric Model
      | 1: Asymetric model
  States : Inport
  Reconf params : Inport  Port=2
  Control Comands : Inport  Port=3
  Acels actual : Scope
      settings: YMin=-0.04  YMax=0.09  SaveName=ScopeData14
  Actuators Dynamcis : Subsystem  TreatAsAtomicUnit=on
  Bus Creator : BusCreator  Inputs=12
  Bus Creator1 : BusCreator  Inputs=2
  Bus Selector : BusSelector  OutputSignals=Blockades,Blockade now,Reconfig signal
  Demux : Demux  Outputs=[13 6]
  Demux1 : Demux  Outputs=8
  F16 nlsim nlplant Asymetrical : MATLABFcn  MATLABFcn=nlplantASYM_Reconf  OutputDimensions=19  OutputSignalType=real
  Fidelity Flag : Constant  Value=fi_flag_Simulink
  Integrate F16 State Derivatives : Integrator  InitialCondition=trim_state
  Leading Edge Flap:Symetric deflection : Subsystem
  Model used flag : Constant  Value=Model_used_flag
  Mux1 : Mux  Inputs=8
  Mux2 : Mux  Inputs=[23 19]
  Mux5 : Mux  Inputs=[13 8 1 1]
  Rotation Angles to Direction Cosine Matrix : aerolibtransform2/Rotation Angles to Direction Cosine Matrix  rotationOrder=ZYX
  Selector : Selector  InputPortWidth=13  Indices=[1:3]
  Selector1 : Selector  InputPortWidth=13  Indices=[1:3]
  Selector2 : Selector  InputPortWidth=13  Indices=[7]
  Selector3 : Selector  InputPortWidth=13  Indices=[8:9]
  Selector4 : Selector  InputPortWidth=13  Indices=[10:12]
  Selector5 : Selector  InputPortWidth=13  Indices=[4:6]
  Selector6 : Selector  InputPortWidth=6  Indices=[1:3]
  Selector7 : Selector  InputPortWidth=3  Indices=[3 2 1]
  Selector9 : Selector  InputPortWidth=13  Indices=[10:12]
  Signal Specification : SignalSpecification  Dimensions=19
  Sum1 : Sum  Inputs=|++  SaturateOnIntegerOverflow=on  InputSameDT=on  OutDataTypeStr=Inherit: Same as first input
  Sum9 : Sum  Inputs=|++  SaturateOnIntegerOverflow=on  InputSameDT=on  OutDataTypeStr=Inherit: Same as first input
  Output_bus : Outport
  Actual control def : Outport  Port=2
  wires:
  Integrate F16 State Derivatives/1 -> Selector5/1, Selector4/1, Selector3/1, Selector2/1, Selector/1, Bus Creator/2  "States_out"
  Rotation Angles to Direction Cosine Matrix/1 -> Bus Creator/10  "DCM_b"
  Bus Creator/1 -> Output_bus/1, Leading Edge Flap:Symetric deflection/1(state)
  Fidelity Flag/1 -> Mux5/3
  Control Comands/1 -> Demux1/1
  States/1 -> Mux5/1
  Mux2/1 -> F16 nlsim nlplant Asymetrical/1  "INPUTS"
  F16 nlsim nlplant Asymetrical/1 -> Demux/1  "OUTPUTS"
  Actuators Dynamcis/2(Dec_Control_def) -> Mux5/2
  Model used flag/1 -> Mux5/4
  Demux1/8 -> Sum1/1
  Demux1/7 -> Sum9/1
  Leading Edge Flap:Symetric deflection/1(delta_lef (deg)) -> Bus Creator1/1, Sum1/2, Sum9/2  "Symetric_LEF_defl"
  Demux1/5 -> Mux1/5
  Demux1/3 -> Mux1/3
  Demux1/1 -> Mux1/1
  Demux1/2 -> Mux1/2
  Demux1/4 -> Mux1/4
  Demux1/6 -> Mux1/6
  Sum9/1 -> Mux1/7
  Sum1/1 -> Mux1/8
  Mux1/1 -> Actuators Dynamcis/1(Control_commands)
  Selector9/1 -> Acels actual/1
  Actuators Dynamcis/3(Throttle_meas) -> Bus Creator/12  "Throttle"
  Demux/1 -> Selector9/1, Bus Creator/1, Selector1/1, Integrate F16 State Derivatives/1  "States_dot_out"
  Selector/1 -> Bus Creator/4  "X_e"
  Selector1/1 -> Bus Creator/5  "V_e"
  Selector2/1 -> Bus Creator/6  "TAS"
  Selector3/1 -> Bus Creator/7  "alpha ; beta"
  Selector4/1 -> Bus Creator/8  "p;q;r"
  Selector5/1 -> Selector7/1, Bus Creator/9  "euler"
  Selector6/1 -> Bus Creator/11  "an_b_CG"
  Demux/2 -> Selector6/1, Bus Creator/3  "Other outs"
  Selector7/1 -> Rotation Angles to Direction Cosine Matrix/1
  Mux5/1 -> Mux2/1  "INPUTS"
  Signal Specification/1 -> Actuators Dynamcis/4(Reconfig signal), Mux2/2
  Reconf params/1 -> Bus Selector/1
  Bus Selector/3 -> Signal Specification/1  "<Reconfig signal>"
  Bus Selector/1 -> Actuators Dynamcis/2(Blockades)  "<Blockades>"
  Bus Selector/2 -> Actuators Dynamcis/3(Blockade now)  "<Blockade now>"
  Bus Creator1/1 -> Actual control def/1
  Actuators Dynamcis/1(Control Defl Plot) -> Bus Creator1/2  "actual_control_defl"

== system F16ASYM_Controlled/FlightGear visualization/Flat Earth to LLA ==
  note: Flat Earth to LLA
  Xe : Inport
  altitude0 : Inport  Port=2
  Angle Conversion : aerolibconvert2/Angle Conversion  IU=deg  OU=rad
  Demux2 : Demux  Outputs=2
  Demux6 : Demux  Outputs=[2 1]
  Display : Display
  Flat Earth to LLA : aerolibtransform2/Flat Earth to LLA  units=Metric (MKS)  ptype=Earth (WGS84)  F=1/298.257223563  R=6378137  LL0=[latitude longitude]  psi=0
  Gain : Gain  Gain=-1
  Mux : Mux  Inputs=2
  longitude l : Outport
  latitude mu : Outport  Port=2
  altitude h : Outport  Port=3
  wires:
  Flat Earth to LLA/1 -> Angle Conversion/1
  Demux2/1 -> latitude mu/1  "latitude"
  Demux2/2 -> longitude l/1
  Xe/1 -> Demux6/1
  altitude0/1 -> Flat Earth to LLA/2
  Flat Earth to LLA/2 -> Display/1, altitude h/1  "altitude"
  Angle Conversion/1 -> Demux2/1
  Mux/1 -> Flat Earth to LLA/1
  Demux6/1 -> Mux/1
  Demux6/2 -> Gain/1
  Gain/1 -> Mux/2

== system F16ASYM_Controlled/FlightGear visualization/Mod controls ==
  "7dof " : Inport
  Add : Sum
  Degrees to Radians{1..6} (6 alike) : simulink_extras/Transformations/Degrees to Radians
  Demux : Demux  Outputs=7
  Gain : Gain  Gain=1/2
  Elevator Sym : Outport
  Left flap : Outport  Port=2
  Right flap : Outport  Port=3
  Left LEF : Outport  Port=4
  Right LEF : Outport  Port=5
  Rudder : Outport  Port=6
  wires:
  "7dof "/1 -> Demux/1
  Demux/1 -> Add/1
  Demux/2 -> Add/2
  Add/1 -> Gain/1
  Demux/3 -> Degrees to Radians1/1
  Demux/4 -> Degrees to Radians2/1
  Demux/5 -> Degrees to Radians3/1
  Demux/6 -> Degrees to Radians4/1
  Degrees to Radians2/1 -> Right flap/1
  Degrees to Radians3/1 -> Rudder/1
  Degrees to Radians4/1 -> Left LEF/1
  Degrees to Radians5/1 -> Right LEF/1
  Gain/1 -> Degrees to Radians6/1
  Degrees to Radians1/1 -> Left flap/1
  Demux/7 -> Degrees to Radians5/1
  Degrees to Radians6/1 -> Elevator Sym/1

== system F16ASYM_Controlled/FlightGear visualization/phidot thetadot psidot ==
  pqr : Inport
  phi theta psi : Inport  Port=2
  Concatenate1 : Concatenate  NumInputs=3
  Concatenate2 : Concatenate  NumInputs=3
  SinCos : aerolibobsolete/SinCos
  keep angles in range [-pi pi] : Trigonometry  Operator=atan2
  phidot : Fcn  Expr=u[1]+(u[2]*u[4]+u[3]*u[7])*(u[5]/u[8])
  psidot : Fcn  Expr=(u[2]*u[4]+u[3]*u[7])/u[8]
  thetadot : Fcn  Expr=u[2]*u[7]-u[3]*u[4]
  ptp_earth : Outport
  ptp_dot : Outport  Port=2
  wires:
  SinCos/2 -> Concatenate1/3, keep angles in range [-pi pi]/2
  SinCos/1 -> Concatenate1/2, keep angles in range [-pi pi]/1
  Concatenate2/1 -> ptp_dot/1
  phidot/1 -> Concatenate2/1
  thetadot/1 -> Concatenate2/2
  psidot/1 -> Concatenate2/3
  phi theta psi/1 -> SinCos/1
  pqr/1 -> Concatenate1/1
  Concatenate1/1 -> thetadot/1, phidot/1, psidot/1
  keep angles in range [-pi pi]/1 -> ptp_earth/1
